simulink model "tip_interaction_closedloop_gain_sched"  (R2018b)
settings: Solver=VariableStepAuto  StartTime=0.0  StopTime=trun  RelTol=1e-9  AbsTol=1e-9
values from neighbouring files (symbols this model uses):
  D_I = zpk([0], 1, KI, G_plant.Ts)    [control_design.m]    (also in force_sim.m; force_sim_gain_sched.m)
  KK = 9    [force_sim.m]    (also in force_sim_gain_sched.m = -20)
  kmax = 2    [force_sim_gain_sched.m]
  kmin = .015    (= 0.015)    [force_sim_gain_sched.m]
  ko = 1    [force_sim_gain_sched.m]
  M = 10*1    (= 10)    [control_design.m]    (also in force_sim.m = 4; force_sim_gain_sched.m = 19.4607843137; x_controller_loop_shaping.m = eye(3))
  m2v = 1/v2m    (= 2857142.85714)    [force_sim.m]    (also in force_sim_gain_sched.m)
  params = struct('sigma', sig, 'k', k, 'Q', Q, 'wo', wo,                 'm', m, 'fo', fo, 'ro', ro)    [force_sim.m]    (also in force_sim_gain_sched.m)
  v2m = (7/20)*1e-6    (= 3.5e-07)    [force_sim.m]    (also in force_sim_gain_sched.m)
libraries: cstblocks x4
settings Model: Creator=arnold  LastModifiedBy=arnold
settings SolverCC: AutoScaleAbsTol=off
settings DebuggingCC: LibraryContextMissingDiagnostic=none
settings SFSimCC: SimUseLocalCustomCode=off
settings RTWCC: RTWUseLocalCustomCode=off
settings CodeAppCC: StateflowObjectComments=on

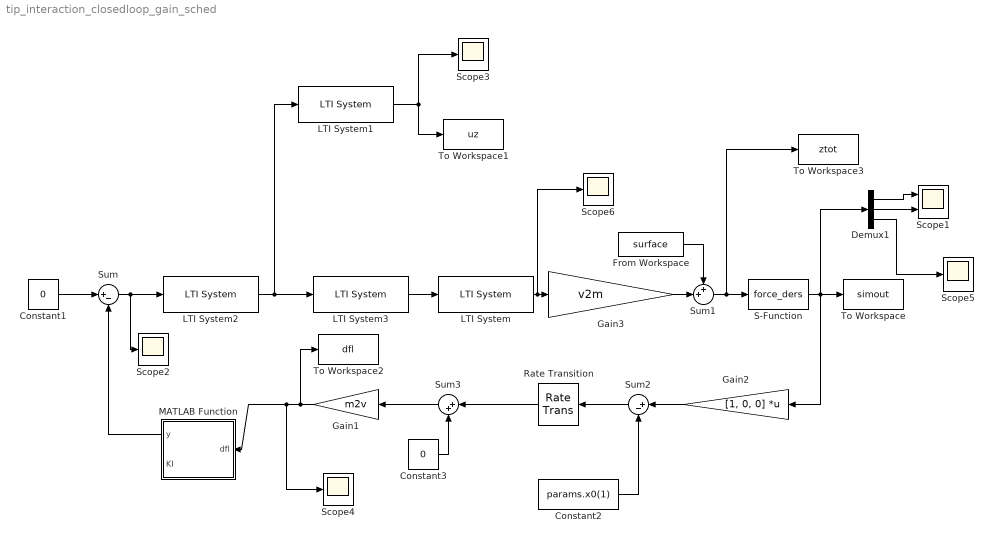
== system tip_interaction_closedloop_gain_sched ==
  Constant1 : Constant  Value=0
  Constant2 : Constant  Value=params.x0(1)
  Constant3 : Constant  Value=0
  Demux1 : Demux  Outputs=3
  From Workspace : FromWorkspace  VariableName=surface  SampleTime=0
  Gain1 : Gain  Gain=m2v
  Gain2 : Gain  Gain=[1, 0, 0]  Multiplication=Matrix(K*u)
  Gain3 : Gain  Gain=v2m
  LTI System : cstblocks/LTI System  sys=G_plant  IC=xss
  LTI System1 : cstblocks/LTI System  sys=models.modelFit.gdrift  IC=xss
  LTI System2 : cstblocks/LTI System  sys=D_I*KK  IC=[]
  LTI System3 : cstblocks/LTI System  sys=models.modelFit.Dinv  IC=xss
  MATLAB Function : MATLAB Function  TreatAsAtomicUnit=on
  Rate Transition : RateTransition  OutPortSampleTime=Ts
  S-Function : S-Function  FunctionName=force_ders  Parameters=params  SFunctionDeploymentMode=off  EnableBusSupport=off
  Scope1 : Scope  NumInputPorts=2
  Scope{2..6} (5 alike) : Scope
  Sum : Sum  Inputs=|+-
  Sum1 : Sum  Inputs=++|
  Sum2 : Sum  Inputs=|+-
  Sum3 : Sum  Inputs=|++
  To Workspace : ToWorkspace  VariableName=simout  SaveFormat=Timeseries  SampleTime=-1
  To Workspace1 : ToWorkspace  VariableName=uz  SaveFormat=Timeseries  SampleTime=-1
  To Workspace2 : ToWorkspace  VariableName=dfl  SaveFormat=Timeseries  SampleTime=-1
  To Workspace3 : ToWorkspace  VariableName=ztot  SaveFormat=Timeseries  SampleTime=-1
  wires:
  Constant1/1 -> Sum/1
  Sum1/1 -> To Workspace3/1, S-Function/1
  Sum/1 -> Scope2/1, LTI System2/1
  LTI System2/1 -> LTI System3/1, LTI System1/1
  LTI System/1 -> Scope6/1, Gain3/1
  S-Function/1 -> Gain2/1, Demux1/1, To Workspace/1
  Demux1/1 -> Scope1/1
  Demux1/2 -> Scope1/2
  Demux1/3 -> Scope5/1
  Gain2/1 -> Sum2/1
  Constant2/1 -> Sum2/2
  Sum2/1 -> Rate Transition/1
  Gain3/1 -> Sum1/2
  LTI System1/1 -> To Workspace1/1, Scope3/1
  LTI System3/1 -> LTI System/1
  Sum3/1 -> Gain1/1
  From Workspace/1 -> Sum1/1
  Gain1/1 -> Scope4/1, MATLAB Function/1(dfl), To Workspace2/1
  MATLAB Function/1(y) -> Sum/2
  Constant3/1 -> Sum3/2
  Rate Transition/1 -> Sum3/1

== matlab function tip_interaction_closedloop_gain_sched/MATLAB Function ==
  data: dfl input; y output; kmax parameter; kmin parameter; ko parameter; M parameter; KI output
function [y, KI] = fcn(dfl, kmax, kmin, ko, M)
  
%   KI = fcn(dfl, kmax, kmin, ko, M)


%   if dfl < -0.01
%     KI = 1*dfl;
%   elseif dfl > 0.01
%     KI = 1*dfl;
%   else
%     KI = dfl;
%   end


KI = ko + M * dfl;
y = KI*dfl;
% KI = min(max(KI, kmin), kmax);
  
end
